simulink model "SolvingODE_Simulink"  (R2024a)
settings: Solver=VariableStepAuto  StartTime=0.0  StopTime=20  FixedStep=0.001  MaxStep=0.001  RelTol=1e-3
undefined symbols (not defined in the file): a, At, C, C0, CA0, CAin, Cin, cp, F, g, h, h0, hA, i0, k, K, L, m, mu, q1, q2, Qin, r, R, T0, tau, theta1, theta2, Tinf, u0, V, Vc0, Vin, x0, y0, y1, y2
settings Model: Creator=buttrakd  LastModifiedBy=buttrakd

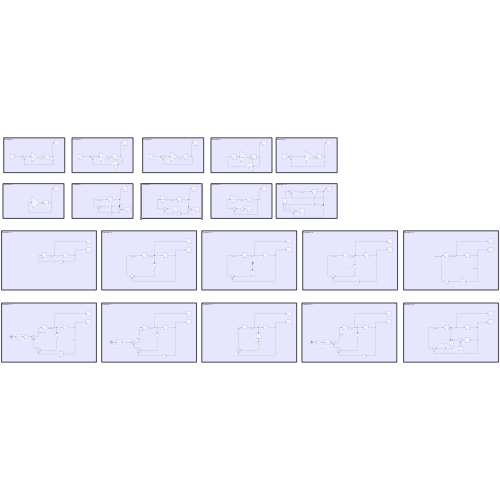
[thumbnail: Simulink's stored preview of the top-level diagram]
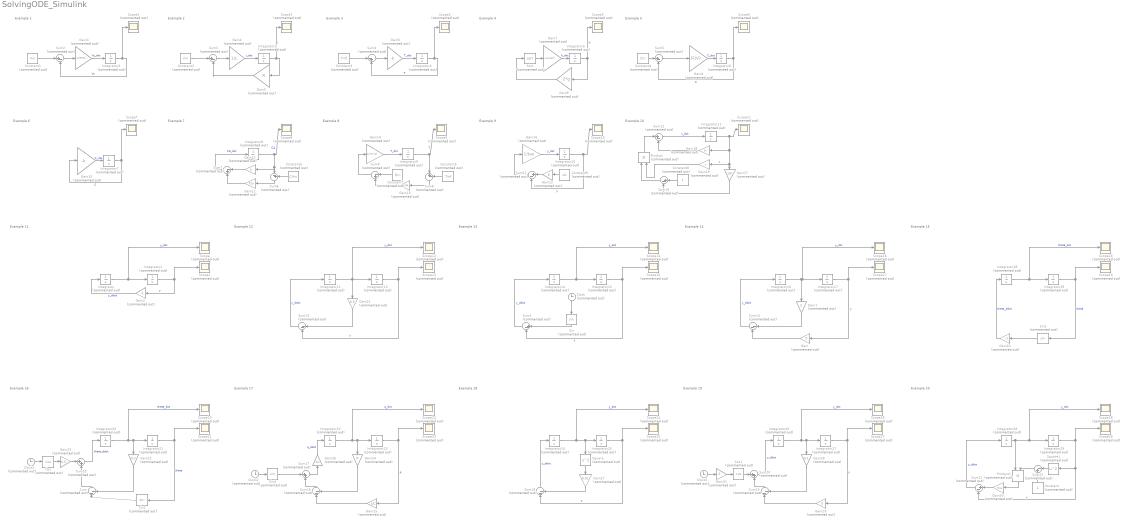
== system SolvingODE_Simulink ==
  note: Example 11
  note: Example 1
  note: Example 2
  note: Example 3
  note: Example 4
  note: Example 5
  note: Example 6
  note: Example 7
  note: Example 8
  note: Example 9
  note: Example 10
  note: Example 12
  note: Example 13
  note: Example 14
  note: Example 15
  note: Example 16
  note: Example 17
  note: Example 18
  note: Example 19
  note: Example 20
  Clock{,1..3} (4 alike) : Clock  Commented=on
  Constant : Constant  Commented=on
  Constant1 : Constant  Commented=on  Value=Vin
  Constant2 : Constant  Commented=on  Value=Vin
  Constant3 : Constant  Commented=on  Value=Tinf
  Constant4 : Constant  Commented=on  Value=Cin
  Constant5 : Constant  Commented=on  Value=CAin
  Constant6 : Constant  Commented=on  Value=Tinf
  Constant7 : Constant  Commented=on  Value=Qin
  Constant8 : Constant  Commented=on
  Constant9 : Constant  Commented=on  Value=u0
  Cos : Trigonometry  Commented=on  Operator=cos
  Cos1 : Trigonometry  Commented=on  Operator=cos
  Gain : Gain  Commented=on  Gain=5
  Gain1 : Gain  Commented=on  Gain=2
  Gain10 : Gain  Commented=on  Gain=-k
  Gain11 : Gain  Commented=on  Gain=F/V
  Gain12 : Gain  Commented=on  Gain=k
  Gain13 : Gain  Commented=on  Gain=hA
  Gain14 : Gain  Commented=on  Gain=1/(m*cp)
  Gain15 : Gain  Commented=on  Gain=K
  Gain16 : Gain  Commented=on  Gain=1/tau
  Gain17 : Gain  Commented=on  Gain=1/K
  Gain18 : Gain  Commented=on  Gain=h
  Gain19 : Gain  Commented=on  Gain=r
  Gain2 : Gain  Commented=on  Gain=-1
  Gain20 : Gain  Commented=on  Gain=-1
  Gain21 : Gain  Commented=on  Gain=0.5
  Gain22 : Gain  Commented=on  Gain=0.2
  Gain23 : Gain  Commented=on  Gain=0.5
  Gain24 : Gain  Commented=on  Gain=R
  Gain25 : Gain  Commented=on  Gain=1/C
  Gain26 : Gain  Commented=on  Gain=1/L
  Gain27 : Gain  Commented=on  Gain=0.01
  Gain28 : Gain  Commented=on  Gain=0.1
  Gain29 : Gain  Commented=on  Gain=3
  Gain3 : Gain  Commented=on  Gain=1/(R*C)
  Gain30 : Gain  Commented=on  Gain=mu
  Gain31 : Gain  Commented=on  Gain=2
  Gain4 : Gain  Commented=on  Gain=1/L
  Gain5 : Gain  Commented=on  Gain=R
  Gain6 : Gain  Commented=on  Gain=-k
  Gain7 : Gain  Commented=on  Gain=-(a/(At))
  Gain8 : Gain  Commented=on  Gain=(F/V)
  Gain9 : Gain  Commented=on  Gain=2*g
  Integrator{,12,14,16,24,26,28} (7 alike) : Integrator  Commented=on  InitialCondition=y2
  Integrator{1,13,15,17,25,27,29} (7 alike) : Integrator  Commented=on  InitialCondition=y1
  Integrator10 : Integrator  Commented=on  InitialCondition=y0
  Integrator11 : Integrator  Commented=on  InitialCondition=x0
  Integrator18 : Integrator  Commented=on  InitialCondition=theta2
  Integrator19 : Integrator  Commented=on  InitialCondition=theta1
  Integrator2 : Integrator  Commented=on  InitialCondition=Vc0
  Integrator20 : Integrator  Commented=on  InitialCondition=theta2
  Integrator21 : Integrator  Commented=on  InitialCondition=theta1
  Integrator22 : Integrator  Commented=on  InitialCondition=q2
  Integrator23 : Integrator  Commented=on  InitialCondition=q1
  Integrator3 : Integrator  Commented=on  InitialCondition=i0
  Integrator4 : Integrator  Commented=on  InitialCondition=T0
  Integrator5 : Integrator  Commented=on  InitialCondition=h0
  Integrator6 : Integrator  Commented=on  InitialCondition=C0
  Integrator7 : Integrator  Commented=on  InitialCondition=CA0
  Integrator8 : Integrator  Commented=on  InitialCondition=CA0
  Integrator9 : Integrator  Commented=on  InitialCondition=T0
  Product : Product  Commented=on
  Product1 : Product  Commented=on
  Scope{,1..29} (30 alike) : Scope  Commented=on
  Sin{,1..2,4} (4 alike) : Trigonometry  Commented=on
  Sqrt : Sqrt  Commented=on
  Square : Math  Commented=on  Operator=square
  Square1 : Math  Commented=on  Operator=square
  Sum{,13..14,16,18..19} (6 alike) : Sum  Commented=on  Inputs=|--
  Sum{1..3,5,8,10..12,21} (9 alike) : Sum  Commented=on  Inputs=|+-
  Sum15 : Sum  Commented=on  Inputs=|++
  Sum17 : Sum  Commented=on  Inputs=|++
  Sum20 : Sum  Commented=on  Inputs=|++
  Sum{4,6..7,9,22} (5 alike) : Sum  Commented=on  Inputs=|-+
  wires:
  Integrator1/1 -> Gain2/1, Scope1/1  "y"
  Integrator/1 -> Scope/1, Integrator1/1  "y_dot"
  Integrator2/1 -> Scope2/1, Sum2/2  "Vc"
  Sum2/1 -> Gain3/1
  Constant1/1 -> Sum2/1
  Gain3/1 -> Integrator2/1  "Vc_dot"
  Gain4/1 -> Integrator3/1  "i_dot"
  Constant2/1 -> Sum3/1
  Sum3/1 -> Gain4/1
  Integrator3/1 -> Gain5/1, Scope3/1  "i"
  Gain5/1 -> Sum3/2
  Integrator4/1 -> Scope4/1, Sum4/2  "T"
  Sum4/1 -> Gain6/1
  Constant3/1 -> Sum4/1
  Gain6/1 -> Integrator4/1  "T_dot"
  Integrator5/1 -> Gain9/1, Scope5/1  "h"
  Gain9/1 -> Sqrt/1
  Sqrt/1 -> Gain7/1
  Gain7/1 -> Integrator5/1  "h_dot"
  Gain8/1 -> Integrator6/1  "C_dot"
  Integrator6/1 -> Sum5/2, Scope6/1  "C"
  Constant4/1 -> Sum5/1
  Sum5/1 -> Gain8/1
  Integrator7/1 -> Gain10/1, Scope7/1  "C"
  Gain10/1 -> Integrator7/1  "C_dot"
  Integrator8/1 -> Scope8/1, Gain12/1, Sum6/1  "CA"
  Constant5/1 -> Sum6/2
  Sum6/1 -> Gain11/1
  Gain11/1 -> Sum7/2
  Gain12/1 -> Sum7/1
  Sum7/1 -> Integrator8/1  "CA_dot"
  Sum9/1 -> Gain14/1
  Gain13/1 -> Sum9/2
  Sum8/1 -> Gain13/1
  Constant6/1 -> Sum8/2
  Integrator9/1 -> Sum8/1, Scope9/1  "T"
  Constant7/1 -> Sum9/1
  Gain14/1 -> Integrator9/1  "T_dot"
  Gain16/1 -> Integrator10/1  "y_dot"
  Constant9/1 -> Gain15/1
  Integrator10/1 -> Sum11/2, Scope10/1  "y"
  Sum11/1 -> Gain16/1
  Gain15/1 -> Sum11/1
  Integrator11/1 -> Scope11/1, Gain18/1, Gain19/1, Gain17/1  "x"
  Sum12/1 -> Integrator11/1  "x_dot"
  Gain17/1 -> Sum10/2
  Constant8/1 -> Sum10/1
  Sum10/1 -> Product/1
  Gain19/1 -> Product/2
  Product/1 -> Sum12/1
  Gain18/1 -> Sum12/2
  Gain21/1 -> Sum13/1
  Integrator13/1 -> Sum13/2, Scope13/1  "y"
  Integrator12/1 -> Integrator13/1, Gain21/1, Scope12/1  "y_dot"
  Sum13/1 -> Integrator12/1  "y_ddot"
  Sum1/1 -> Integrator14/1  "y_ddot"
  Integrator14/1 -> Scope14/1, Integrator15/1  "y_dot"
  Integrator15/1 -> Scope15/1, Sum1/2  "y"
  Sin/1 -> Sum1/1
  Clock/1 -> Sin/1
  Integrator17/1 -> Gain/1, Scope17/1  "y"
  Integrator16/1 -> Integrator17/1, Scope16/1, Gain1/1  "y_dot"
  Sum14/1 -> Integrator16/1  "y_ddot"
  Gain/1 -> Sum14/2
  Gain1/1 -> Sum14/1
  Gain20/1 -> Integrator18/1  "theta_ddot"
  Integrator18/1 -> Scope18/1, Integrator19/1  "theta_dot"
  Integrator19/1 -> Scope19/1, Sin1/1  "theta"
  Sin1/1 -> Gain20/1
  Sin2/1 -> Sum/1
  Integrator21/1 -> Sin2/1, Scope21/1  "theta"
  Integrator20/1 -> Integrator21/1, Gain22/1, Scope20/1  "theta_dot"
  Gain22/1 -> Sum/2
  Sum/1 -> Sum15/2
  Clock1/1 -> Cos/1
  Cos/1 -> Gain23/1
  Gain23/1 -> Sum15/1
  Sum15/1 -> Integrator20/1  "theta_ddot"
  Sum17/1 -> Gain26/1
  Sin4/1 -> Sum17/1
  Clock2/1 -> Sin4/1
  Sum16/1 -> Sum17/2
  Gain24/1 -> Sum16/2
  Integrator22/1 -> Scope22/1, Gain24/1, Integrator23/1  "q_dot"
  Integrator23/1 -> Gain25/1, Scope23/1  "q"
  Gain25/1 -> Sum16/1
  Gain26/1 -> Integrator22/1  "q_ddot"
  Sum18/1 -> Integrator24/1  "y_ddot"
  Integrator25/1 -> Sum18/1, Scope25/1  "y"
  Integrator24/1 -> Integrator25/1, Square/1, Scope24/1  "y_dot"
  Gain27/1 -> Sum18/2
  Square/1 -> Gain27/1
  Sum20/1 -> Integrator26/1  "y_ddot"
  Gain29/1 -> Sum19/1
  Integrator27/1 -> Scope27/1, Gain29/1  "y"
  Integrator26/1 -> Integrator27/1, Gain28/1, Scope26/1  "y_dot"
  Gain28/1 -> Sum19/2
  Sum19/1 -> Sum20/2
  Clock3/1 -> Gain31/1
  Cos1/1 -> Sum20/1
  Gain31/1 -> Cos1/1
  Sum21/1 -> Integrator28/1  "y_ddot"
  Integrator28/1 -> Integrator29/1, Scope28/1, Product1/1  "y_dot"
  Integrator29/1 -> Square1/1, Sum21/2, Scope29/1  "y"
  Constant/1 -> Sum22/2
  Square1/1 -> Sum22/1
  Sum22/1 -> Product1/2
  Product1/1 -> Gain30/1
  Gain30/1 -> Sum21/1
  Gain2/1 -> Integrator/1  "y_ddot"
